simulink model "MOTOR"  (R2021b)
settings: Solver=FixedStepDiscrete  StartTime=0.0  StopTime=10.0  FixedStep=0.001  RelTol=1e-3
libraries: GPIO_Lib x2, USART_Lib x2, STM32_Config_Lib x1, TIMERS_Lib x1
settings Model: Creator=Daniel  LastModifiedBy=Daniel
settings OptimizationCC: DefaultParameterBehavior=Inlined  EnhancedBackFolding=on  PassReuseOutputArgsAs=Individual arguments  ZeroExternalMemoryAtStartup=off  ZeroInternalMemoryAtStartup=off  OptimizeBlockOrder=speed  DifferentSizesBufferReuse=on  OptimizationCustomize=off  EfficientTunableParamExpr=on
settings DebuggingCC: ParameterTunabilityLossMsg=error
settings SFSimCC: MATLABDynamicMemAlloc=off
settings RTWCC: Description=stm32 (Embedded Target)  SystemTargetFile=stm32.tlc  TemplateMakefile=stm32.tmf  GenerateReport=on
settings CodeAppCC: ForceParamTrailComments=on  IgnoreCustomStorageClasses=off  MaxIdLength=64  OperatorAnnotations=on  SimulinkDataObjDesc=on  SFDataObjDesc=on  CustomSymbolStrType=$N$R$M  StateflowObjectComments=on  MATLABSourceComments=on
settings STFCustomTargetCC: TargetLangStandard=C99 (ISO)  CodeReplacementLibrary=ARM CMSIS SIN COS  MultiwordLength=256  ParMdlRefBuildCompliant=on  IncludeMdlTerminateFcn=off  CombineOutputUpdateFcns=on  ERTCustomFileBanners=on  SupportContinuousTime=off  SupportNonInlinedSFcns=off  RemoveResetFunc=on  MATLABClassNameForMDSCustomization=Simulink.SoftwareTarget.ERTCustomization  GRTInterface=off  SystemTargetFile=stm32.tlc
settings ERTTargetCC: TargetLangStandard=C99 (ISO)  CodeReplacementLibrary=ARM CMSIS SIN COS  CompOptLevelCompliant=off  ConcurrentExecutionCompliant=off  IncludeMdlTerminateFcn=off  ModelStepFunctionPrototypeControlCompliant=off  CPPClassGenCompliant=off  UseToolchainInfoCompliant=off  ExtModeStaticAllocSize=256  ExtModeMexFile=ext_serial_win32_comm  ExtModeMexArgs=0,1,115200,10  InlinedParameterPlacement=NonHierarchical  ERTSrcFileBannerTemplate=sourceFileTemplate.cgt  ERTHdrFileBannerTemplate=sourceFileTemplate.cgt  ERTDataSrcFileTemplate=sourceFileTemplate.cgt  ERTDataHdrFileTemplate=sourceFileTemplate.cgt  ERTCustomFileTemplate=customRoutineProcess.tlc

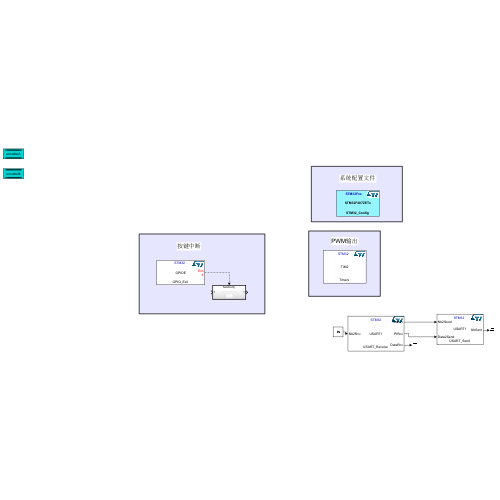
[thumbnail: Simulink's stored preview of the top-level diagram]
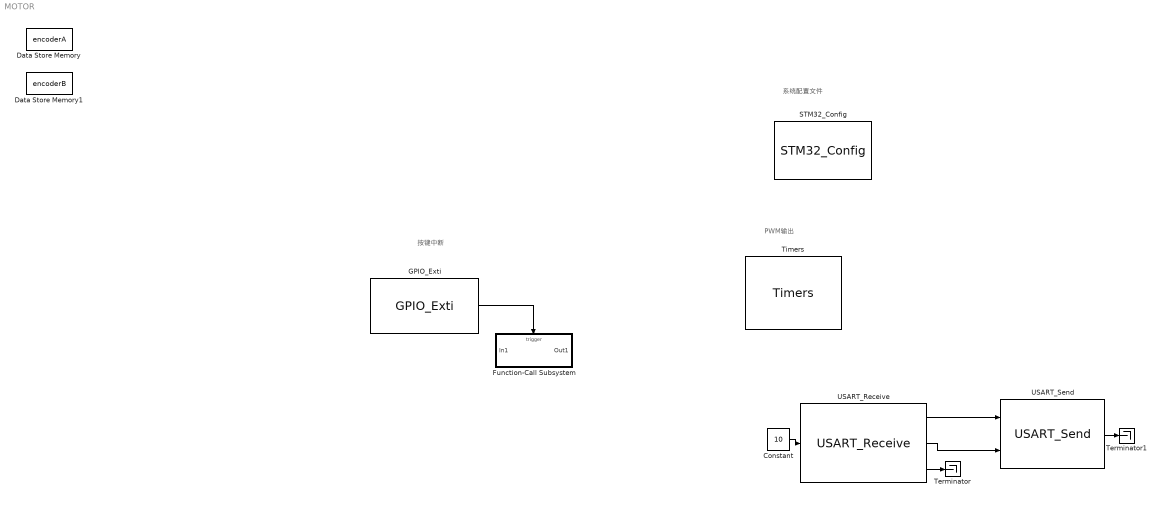
== system MOTOR ==
  note: 按键中断
  note: 系统配置文件
  note: PWM输出
  Constant : Constant  Value=10  OutDataTypeStr=uint16
  Data Store Memory : DataStoreMemory  DataStoreName=encoderA  ReadBeforeWriteMsg=warning  WriteAfterWriteMsg=warning  WriteAfterReadMsg=warning  ShowAdditionalParam=off
  Data Store Memory1 : DataStoreMemory  DataStoreName=encoderB  ReadBeforeWriteMsg=warning  WriteAfterWriteMsg=warning  WriteAfterReadMsg=warning  ShowAdditionalParam=off
  Function-Call Subsystem : Subsystem  TreatAsAtomicUnit=on
  GPIO_Exti : GPIO_Lib/GPIO_Exti  Port_name=GPIOE  Pin_0=off  Pin_1=off  Pin_2=off  Pin_3=off  Pin_4=on  Pin_5=off  Pin_6=off  Pin_7=off  Pin_8=off  Pin_9=off  Pin_10=off  Pin_11=off  Pin_12=off  Pin_13=off  Pin_14=off  Pin_15=off  PinList=GPIOE4
      settings: SourceProductName=Target Support Package - STM32 Adapter
  STM32_Config : STM32_Config_Lib/STM32_Config  Priority=0  Project_Path=.\  Config_File=MOTOR.ioc  MCU_Name=STM32F407ZETx
      settings: SourceProductName=Target Support Package - STM32 Adapter
  Terminator : Terminator
  Terminator1 : Terminator
  Timers : TIMERS_Lib/Timers  currentTIM=TIM2  TIM_Name=TIM2  sysUsingTimer=off  TIM_APBClock=72000000  TIM_Set_Clk=off  TIM_Prescaler=71  TIM_Clock=1000000.00  Variable_frequency=off  TIM_Set_OutFreq=on  TIM_ARR=1000  Output_frequency=1000.00  Repetition_counter=0  TIM_Mode=Up  TIM_DMA=none  TIM_IRQ=off  TIM_IRQ_ONLY=off  TIM_UP=off  TIM_TRG=off  TIM_COM=off  TIM_BRK=off  NbTIM=1  CH1_enable=off  CH1N_enable=off  CH1_type=Unknown  CH1_DMA=off  CH1_int=off  CH1_edge=Rising  CH1_div=1  CH1_variable_duty=off  CH1_set_pulse=off  CH1_output_duty=0.00  CH1_pulse=0  CH2_enable=off  CH2N_enable=off  CH2_type=Unknown  CH2_DMA=off  CH2_int=off  CH2_edge=Rising  CH2_div=1  CH2_variable_duty=off  CH2_set_pulse=off  CH2_output_duty=0.00  CH2_pulse=0  CH3_enable=on  CH3N_enable=off  CH3_type=Output_PWM  CH3_DMA=off  CH3_int=off  CH3_edge=Rising  CH3_div=1  CH3_variable_duty=off  CH3_set_pulse=off  CH3_output_duty=50.00  CH3_pulse=500  CH4_enable=off  CH4N_enable=off  CH4_type=Unknown  CH4_DMA=off  CH4_int=off  CH4_edge=Rising  CH4_div=1  CH4_variable_duty=off  CH4_set_pulse=off  CH4_output_duty=0.00  CH4_pulse=0
      settings: SourceProductName=Target Support Package - STM32 Adapter
  USART_Receive : USART_Lib/USART_Receive  USART_name=USART1  Buff_size=512  nbUsart=1  Soft_it=off  Soft_num=0  usartMode=Asynchronous  usartDma_Rx=off  usartDma_Tx=off  usartIt=on
      settings: SourceProductName=Target Support Package - STM32 Adapter
  USART_Send : USART_Lib/USART_Send  USART_name=USART1  Buff_size=512  nbUsart=1  usartMode=Asynchronous  usartDma_Rx=off  usartDma_Tx=off  usartIt=on
      settings: SourceProductName=Target Support Package - STM32 Adapter
  wires:
  GPIO_Exti/1 -> Function-Call Subsystem/Trigger
  USART_Receive/2 -> USART_Send/2
  USART_Receive/3 -> Terminator/1
  Constant/1 -> USART_Receive/1
  USART_Receive/1 -> USART_Send/1
  USART_Send/1 -> Terminator1/1

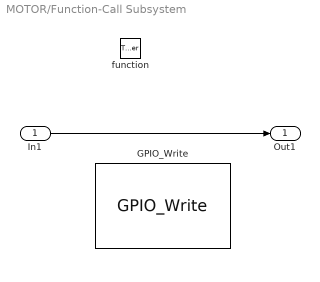
== system MOTOR/Function-Call Subsystem ==
  In1 : Inport
  function : TriggerPort  TriggerType=function-call  VariantControl=(inherit)
  GPIO_Write : GPIO_Lib/GPIO_Write  Port_name=GPIOA  Pin0=off  Toggle_Pin0=off  Pin1=off  Toggle_Pin1=off  Pin2=off  Toggle_Pin2=off  Pin3=off  Toggle_Pin3=off  Pin4=on  Toggle_Pin4=on  Pin5=on  Toggle_Pin5=on  Pin6=off  Toggle_Pin6=off  Pin7=off  Toggle_Pin7=off  Pin8=off  Toggle_Pin8=off  Pin9=off  Toggle_Pin9=off  Pin10=off  Toggle_Pin10=off  Pin11=off  Toggle_Pin11=off  Pin12=off  Toggle_Pin12=off  Pin13=off  Toggle_Pin13=off  Pin14=off  Toggle_Pin14=off  Pin15=off  Toggle_Pin15=off  PinList="GPIOA4  5"
      settings: SourceProductName=Target Support Package - STM32 Adapter
  Out1 : Outport
  wires:
  In1/1 -> Out1/1
